simulink model "TJunctionPrototype"  (R2021a)
settings: Solver=VariableStepAuto  StartTime=0.0  StopTime=10.0  RelTol=1e-3
undefined symbols (not defined in the file): Rk
libraries: EdgesLibrary x8, StreetLanesLibrary x6
settings Model: Creator=phill  LastModifiedBy=phill

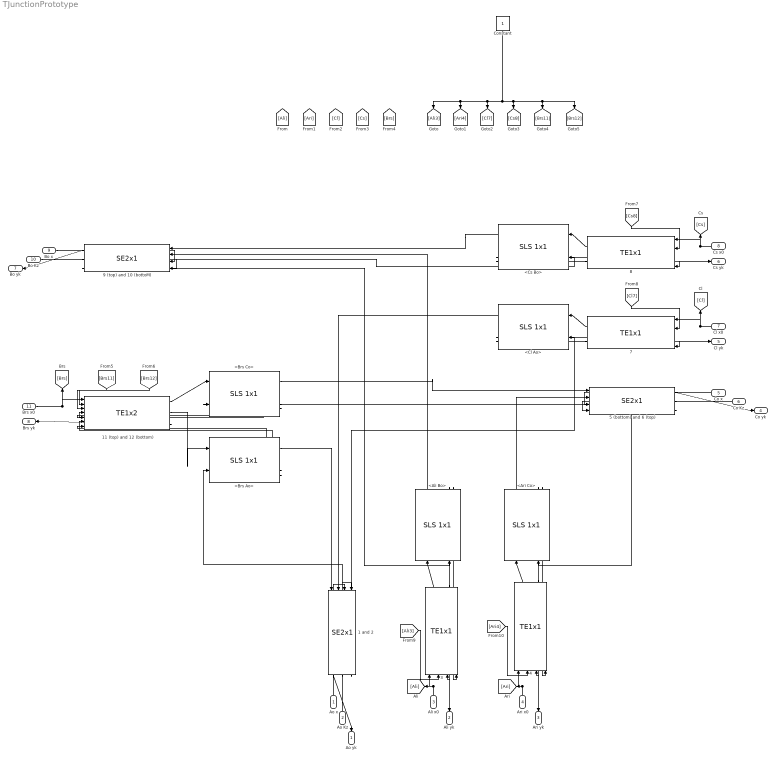
== system TJunctionPrototype ==
  Ao x : Inport
  Ao Kz : Inport  Port=2
  Ali x0 : Inport  Port=3
  Ari x0 : Inport  Port=4
  Co x : Inport  Port=5
  Co Kz : Inport  Port=6
  Cl x0 : Inport  Port=7
  Cs x0 : Inport  Port=8
  Bo x : Inport  Port=9
  Bo Kz : Inport  Port=10
  Brs x0 : Inport  Port=11
  1 and 2 : EdgesLibrary/SE2x1  Rk1=Rk  Rk2=Rk
  11 (top) and 12 (bottom) : EdgesLibrary/TE1x2  Rk1=0.5*Rk  Rk2=0.5*Rk
  {3..4,7..8} (4 alike) : EdgesLibrary/TE1x1  Rk=Rk
  5 (bottom) and 6 (top) : EdgesLibrary/SE2x1  Rk1=Rk*0.5  Rk2=Rk*0.5
  9 (top) and 10 (bottoM) : EdgesLibrary/SE2x1  Rk1=Rk  Rk2=Rk
  <Ali Bo> : StreetLanesLibrary/SLS 1x1  Kz=Kz_left  Tz=Tz_left
  <Ari Co> : StreetLanesLibrary/SLS 1x1  Kz=Kz_right  Tz=Tz_right
  <Brs Ao> : StreetLanesLibrary/SLS 1x1  Kz=Kz_right  Tz=Tz_right
  <Brs Co> : StreetLanesLibrary/SLS 1x1  Kz=Kz_straight  Tz=Tz_straight
  <Cl Ao> : StreetLanesLibrary/SLS 1x1  Kz=Kz_left  Tz=Tz_left
  <Cs Bo> : StreetLanesLibrary/SLS 1x1  Kz=Kz_straight  Tz=Tz_straight
  Constant : Constant  OutDataTypeStr=boolean
  Ao yk : Outport
  Ali yk : Outport  Port=2
  Ari yk : Outport  Port=3
  Co yk : Outport  Port=4
  Cl yk : Outport  Port=5
  Cs yk : Outport  Port=6
  Bo yk : Outport  Port=7
  Brs yk : Outport  Port=8
  wires:
  <Brs Co>/2 -> 5 (bottom) and 6 (top)/1
  5 (bottom) and 6 (top)/2 -> <Brs Co>/2
  <Brs Co>/7 -> 11 (top) and 12 (bottom)/4
  <Brs Co>/8 -> 11 (top) and 12 (bottom)/5
  11 (top) and 12 (bottom)/1 -> <Brs Co>/1
  <Brs Ao>/7 -> 11 (top) and 12 (bottom)/6
  <Brs Ao>/8 -> 11 (top) and 12 (bottom)/7
  11 (top) and 12 (bottom)/2 -> <Brs Ao>/1
  1 and 2/2 -> <Brs Ao>/2
  <Brs Ao>/2 -> 1 and 2/1
  7/1 -> <Cl Ao>/1
  <Cl Ao>/8 -> 7/4
  <Cl Ao>/7 -> 7/3
  8/1 -> <Cs Bo>/1
  <Cs Bo>/8 -> 8/4
  <Cs Bo>/7 -> 8/3
  <Ali Bo>/7 -> 3/3
  <Ali Bo>/8 -> 3/4
  3/1 -> <Ali Bo>/1
  <Ari Co>/7 -> 4/3
  <Ari Co>/8 -> 4/4
  4/1 -> <Ari Co>/1
  5 (bottom) and 6 (top)/3 -> <Ari Co>/2
  <Ari Co>/2 -> 5 (bottom) and 6 (top)/2
  <Cs Bo>/2 -> 9 (top) and 10 (bottoM)/1
  9 (top) and 10 (bottoM)/2 -> <Cs Bo>/2
  <Ali Bo>/2 -> 9 (top) and 10 (bottoM)/2
  9 (top) and 10 (bottoM)/3 -> <Ali Bo>/2
  1 and 2/3 -> <Cl Ao>/2
  <Cl Ao>/2 -> 1 and 2/2
  Ao x/1 -> 1 and 2/3
  Ao Kz/1 -> 1 and 2/4
  1 and 2/1 -> Ao yk/1
  Ali x0/1 -> [Ali], 3/1
  3/2 -> Ali yk/1
  Ari x0/1 -> [Ari], 4/1
  4/2 -> Ari yk/1
  Co x/1 -> 5 (bottom) and 6 (top)/3
  Co Kz/1 -> 5 (bottom) and 6 (top)/4
  5 (bottom) and 6 (top)/1 -> Co yk/1
  Cl x0/1 -> [Cl], 7/1
  7/2 -> Cl yk/1
  Cs x0/1 -> [Cs], 8/1
  8/2 -> Cs yk/1
  Bo x/1 -> 9 (top) and 10 (bottoM)/3
  Bo Kz/1 -> 9 (top) and 10 (bottoM)/4
  9 (top) and 10 (bottoM)/1 -> Bo yk/1
  Brs x0/1 -> 11 (top) and 12 (bottom)/1, [Brs]
  11 (top) and 12 (bottom)/3 -> Brs yk/1
  [Brs11] -> 11 (top) and 12 (bottom)/2
  [Brs12] -> 11 (top) and 12 (bottom)/3
  [Cs8] -> 8/2
  [Cl7] -> 7/2
  [Ali3] -> 3/2
  [Ari4] -> 4/2
  Constant/1 -> [Ari4], [Ali3], [Cl7], [Brs12], [Brs11], [Cs8]
